simulink model "SF020_SysFaultMngt"  (R2022b)
settings: configuration reference "ASW_Configuration_Set_5ms" (kept outside this file)
settings Model: DataDictionary=SF020_SysFaultMngt.sldd  Creator=donglx1  LastModifiedBy=donglx1
settings ConfigSetRef: SourceName=ASW_Configuration_Set_5ms

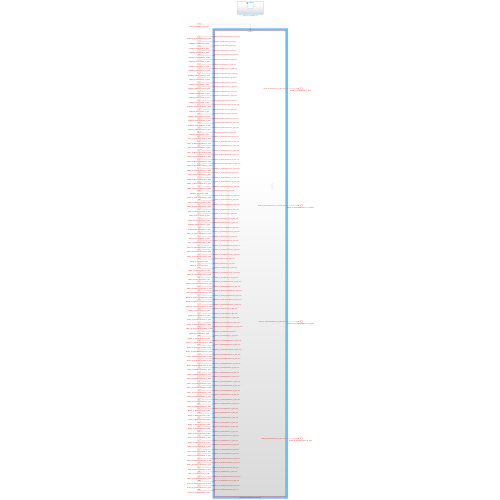
[thumbnail: Simulink's stored preview of the top-level diagram]
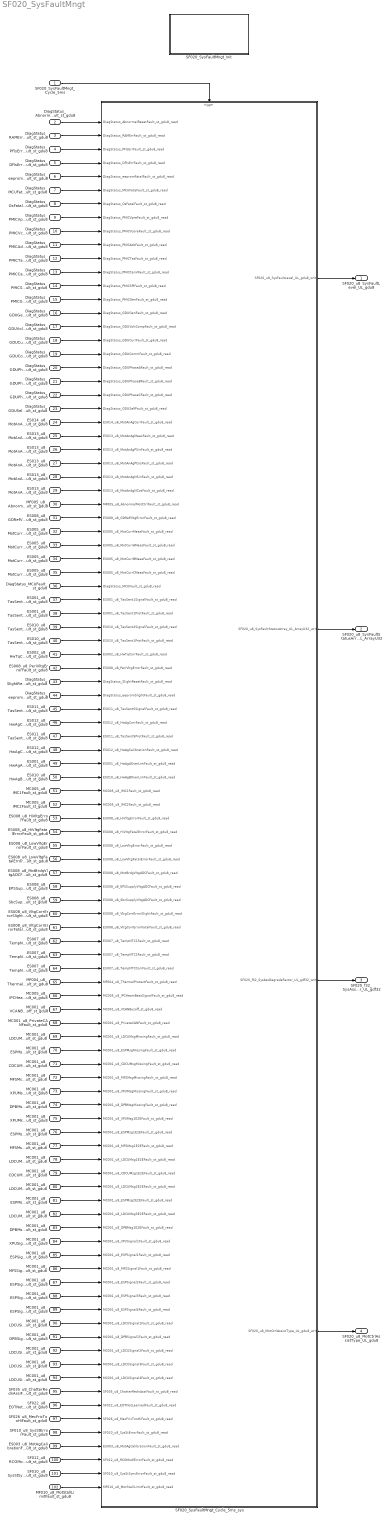
== system SF020_SysFaultMngt ==
  SF020_SysFaultMngt_Cycle_5ms : Inport  SampleTime=0.005  OutputFunctionCall=on
  DiagStatus_AbnormalResetFault_st_gdu8 : Inport  Port=2  OutDataTypeStr=UINT8  PortDimensions=1
  DiagStatus_RAMErrFault_st_gdu8 : Inport  Port=3  OutDataTypeStr=UINT8  PortDimensions=1
  DiagStatus_PFlsErrFault_st_gdu8 : Inport  Port=4  OutDataTypeStr=UINT8  PortDimensions=1
  DiagStatus_DFlsErrFault_st_gdu8 : Inport  Port=5  OutDataTypeStr=UINT8  PortDimensions=1
  DiagStatus_eepromFatalFault_st_gdu8 : Inport  Port=6  OutDataTypeStr=UINT8  PortDimensions=1
  DiagStatus_MCUFataFault_st_gdu8 : Inport  Port=7  OutDataTypeStr=UINT8  PortDimensions=1
  DiagStatus_OsFatalFault_st_gdu8 : Inport  Port=8  OutDataTypeStr=UINT8  PortDimensions=1
  DiagStatus_PMICVpreFault_st_gdu8 : Inport  Port=9  OutDataTypeStr=UINT8  PortDimensions=1
  DiagStatus_PMICVcoreFault_st_gdu8 : Inport  Port=10  OutDataTypeStr=UINT8  PortDimensions=1
  DiagStatus_PMICAdcFault_st_gdu8 : Inport  Port=11  OutDataTypeStr=UINT8  PortDimensions=1
  DiagStatus_PMICTasFault_st_gdu8 : Inport  Port=12  OutDataTypeStr=UINT8  PortDimensions=1
  DiagStatus_PMICCanVFault_st_gdu8 : Inport  Port=13  OutDataTypeStr=UINT8  PortDimensions=1
  DiagStatus_PMICSPIFault_st_gdu8 : Inport  Port=14  OutDataTypeStr=UINT8  PortDimensions=1
  DiagStatus_PMICGenFault_st_gdu8 : Inport  Port=15  OutDataTypeStr=UINT8  PortDimensions=1
  DiagStatus_GDUGenFault_st_gdu8 : Inport  Port=16  OutDataTypeStr=UINT8  PortDimensions=1
  DiagStatus_GDUVoltCompFault_st_gdu8 : Inport  Port=17  OutDataTypeStr=UINT8  PortDimensions=1
  DiagStatus_GDUCurrFault_st_gdu8 : Inport  Port=18  OutDataTypeStr=UINT8  PortDimensions=1
  DiagStatus_GDUCommFault_st_gdu8 : Inport  Port=19  OutDataTypeStr=UINT8  PortDimensions=1
  DiagStatus_GDUPhaseAFault_st_gdu8 : Inport  Port=20  OutDataTypeStr=UINT8  PortDimensions=1
  DiagStatus_GDUPhaseBFault_st_gdu8 : Inport  Port=21  OutDataTypeStr=UINT8  PortDimensions=1
  DiagStatus_GDUPhaseCFault_st_gdu8 : Inport  Port=22  OutDataTypeStr=UINT8  PortDimensions=1
  DiagStatus_GDUSelfFault_st_gdu8 : Inport  Port=23  OutDataTypeStr=UINT8  PortDimensions=1
  ES014_u8_MotAnAgCorrFault_st_gdu8 : Inport  Port=24  OutDataTypeStr=UINT8  PortDimensions=1
  ES013_u8_MotAnAgMeasFault_st_gdu8 : Inport  Port=25  OutDataTypeStr=UINT8  PortDimensions=1
  ES013_u8_MotAnAgPSinFault_st_gdu8 : Inport  Port=26  OutDataTypeStr=UINT8  PortDimensions=1
  ES013_u8_MotAnAgPCosFault_st_gdu8 : Inport  Port=27  OutDataTypeStr=UINT8  PortDimensions=1
  ES013_u8_MotAnAgNSinFault_st_gdu8 : Inport  Port=28  OutDataTypeStr=UINT8  PortDimensions=1
  ES013_u8_MotAnAgNCosFault_st_gdu8 : Inport  Port=29  OutDataTypeStr=UINT8  PortDimensions=1
  MF005_u8_AbnormalMotCtrlFault_st_gdu8 : Inport  Port=30  OutDataTypeStr=UINT8  PortDimensions=1
  ES008_u8_GDRefVltgErrorFault_st_gdu8 : Inport  Port=31  OutDataTypeStr=UINT8  PortDimensions=1
  ES005_u8_MotCurrMeasFault_st_gdu8 : Inport  Port=32  OutDataTypeStr=UINT8  PortDimensions=1
  ES005_u8_MotCurrAMeasFault_st_gdu8 : Inport  Port=33  OutDataTypeStr=UINT8  PortDimensions=1
  ES005_u8_MotCurrBMeasFault_st_gdu8 : Inport  Port=34  OutDataTypeStr=UINT8  PortDimensions=1
  ES005_u8_MotCurrCMeasFault_st_gdu8 : Inport  Port=35  OutDataTypeStr=UINT8  PortDimensions=1
  DiagStatus_MCUFault_st_gdu8 : Inport  Port=36  OutDataTypeStr=UINT8  PortDimensions=1
  ES001_u8_TasSent1SignalFault_st_gdu8 : Inport  Port=37  OutDataTypeStr=UINT8  PortDimensions=1
  ES001_u8_TasSent1ProtFault_st_gdu8 : Inport  Port=38  OutDataTypeStr=UINT8  PortDimensions=1
  ES010_u8_TasSent2SignalFault_st_gdu8 : Inport  Port=39  OutDataTypeStr=UINT8  PortDimensions=1
  ES010_u8_TasSent1ProtFault_st_gdu8 : Inport  Port=40  OutDataTypeStr=UINT8  PortDimensions=1
  ES002_u8_HwTqCorrFault_st_gdu8 : Inport  Port=41  OutDataTypeStr=UINT8  PortDimensions=1
  ES008_u8_PeriVltgErrorFault_st_gdu8 : Inport  Port=42  OutDataTypeStr=UINT8  PortDimensions=1
  DiagStatus_SlightResetFault_st_gdu8 : Inport  Port=43  OutDataTypeStr=UINT8  PortDimensions=1
  DiagStatus_eepromSlightFault_st_gdu8 : Inport  Port=44  OutDataTypeStr=UINT8  PortDimensions=1
  ES011_u8_TasSent5SignalFault_st_gdu8 : Inport  Port=45  OutDataTypeStr=UINT8  PortDimensions=1
  ES012_u8_HwAgCorrFault_st_gdu8 : Inport  Port=46  OutDataTypeStr=UINT8  PortDimensions=1
  ES011_u8_TasSent5ProtFault_st_gdu8 : Inport  Port=47  OutDataTypeStr=UINT8  PortDimensions=1
  ES012_u8_HwAgCalibrationFault_st_gdu8 : Inport  Port=48  OutDataTypeStr=UINT8  PortDimensions=1
  ES001_u8_HwAgAOverLimFault_st_gdu8 : Inport  Port=49  OutDataTypeStr=UINT8  PortDimensions=1
  ES010_u8_HwAgBOverLimFault_st_gdu8 : Inport  Port=50  OutDataTypeStr=UINT8  PortDimensions=1
  MC005_u8_IMC1Fault_st_gdu8 : Inport  Port=51  OutDataTypeStr=UINT8  PortDimensions=1
  MC005_u8_IMC2Fault_st_gdu8 : Inport  Port=52  OutDataTypeStr=UINT8  PortDimensions=1
  ES008_u8_HiVltgErrorFault_st_gdu8 : Inport  Port=53  OutDataTypeStr=UINT8  PortDimensions=1
  ES008_u8_HiVltgFatalErrorFault_st_gdu8 : Inport  Port=54  OutDataTypeStr=UINT8  PortDimensions=1
  ES008_u8_LowVltgErrorFault_st_gdu8 : Inport  Port=55  OutDataTypeStr=UINT8  PortDimensions=1
  ES008_u8_LowVltgFatalErrorFault_st_gdu8 : Inport  Port=56  OutDataTypeStr=UINT8  PortDimensions=1
  ES008_u8_MotBrdgVltgADCFault_st_gdu8 : Inport  Port=57  OutDataTypeStr=UINT8  PortDimensions=1
  ES008_u8_EPSSupplyVltgADCFault_st_gdu8 : Inport  Port=58  OutDataTypeStr=UINT8  PortDimensions=1
  ES008_u8_SbcSupplyVltgADCFault_st_gdu8 : Inport  Port=59  OutDataTypeStr=UINT8  PortDimensions=1
  ES008_u8_VltgCorrErrorSlightFault_st_gdu8 : Inport  Port=60  OutDataTypeStr=UINT8  PortDimensions=1
  ES008_u8_VltgCorrErrorFatalFault_st_gdu8 : Inport  Port=61  OutDataTypeStr=UINT8  PortDimensions=1
  ES007_u8_TempNTC1Fault_st_gdu8 : Inport  Port=62  OutDataTypeStr=UINT8  PortDimensions=1
  ES007_u8_TempNTC2Fault_st_gdu8 : Inport  Port=63  OutDataTypeStr=UINT8  PortDimensions=1
  ES007_u8_TempNTCCorrFault_st_gdu8 : Inport  Port=64  OutDataTypeStr=UINT8  PortDimensions=1
  MF004_u8_ThermalProtectFault_st_gdu8 : Inport  Port=65  OutDataTypeStr=UINT8  PortDimensions=1
  MC005_u8_IPCHeartBeatSignalFault_st_gdu8 : Inport  Port=66  OutDataTypeStr=UINT8  PortDimensions=1
  MC001_u8_VCANBusoff_st_gdu8 : Inport  Port=67  OutDataTypeStr=UINT8  PortDimensions=1
  MC001_u8_PrivateCANFault_st_gdu8 : Inport  Port=68  OutDataTypeStr=UINT8  PortDimensions=1
  MC001_u8_LDCUMsgMissingFault_st_gdu8 : Inport  Port=69  OutDataTypeStr=UINT8  PortDimensions=1
  MC001_u8_ESPMsgMissingFault_st_gdu8 : Inport  Port=70  OutDataTypeStr=UINT8  PortDimensions=1
  MC001_u8_CDCUMsgMissingFault_st_gdu8 : Inport  Port=71  OutDataTypeStr=UINT8  PortDimensions=1
  MC001_u8_MFSMsgMissingFault_st_gdu8 : Inport  Port=72  OutDataTypeStr=UINT8  PortDimensions=1
  MC001_u8_XPUMsgMissingFault_st_gdu8 : Inport  Port=73  OutDataTypeStr=UINT8  PortDimensions=1
  MC001_u8_DPBMsgMissingFault_st_gdu8 : Inport  Port=74  OutDataTypeStr=UINT8  PortDimensions=1
  MC001_u8_XPUMsg1E2EFault_st_gdu8 : Inport  Port=75  OutDataTypeStr=UINT8  PortDimensions=1
  MC001_u8_ESPMsg1E2EFault_st_gdu8 : Inport  Port=76  OutDataTypeStr=UINT8  PortDimensions=1
  MC001_u8_MFSMsg1E2EFault_st_gdu8 : Inport  Port=77  OutDataTypeStr=UINT8  PortDimensions=1
  MC001_u8_LDCUMsg1E2EFault_st_gdu8 : Inport  Port=78  OutDataTypeStr=UINT8  PortDimensions=1
  MC001_u8_CDCUMsg1E2EFault_st_gdu8 : Inport  Port=79  OutDataTypeStr=UINT8  PortDimensions=1
  MC001_u8_LDCUMsg2E2EFault_st_gdu8 : Inport  Port=80  OutDataTypeStr=UINT8  PortDimensions=1
  MC001_u8_ESPMsg2E2EFault_st_gdu8 : Inport  Port=81  OutDataTypeStr=UINT8  PortDimensions=1
  MC001_u8_LDCUMsg3E2EFault_st_gdu8 : Inport  Port=82  OutDataTypeStr=UINT8  PortDimensions=1
  MC001_u8_DPBMsg1E2EFault_st_gdu8 : Inport  Port=83  OutDataTypeStr=UINT8  PortDimensions=1
  MC001_u8_XPUSignal1Fault_st_gdu8 : Inport  Port=84  OutDataTypeStr=UINT8  PortDimensions=1
  MC001_u8_ESPSignal1Fault_st_gdu8 : Inport  Port=85  OutDataTypeStr=UINT8  PortDimensions=1
  MC001_u8_MFSSignal1Fault_st_gdu8 : Inport  Port=86  OutDataTypeStr=UINT8  PortDimensions=1
  MC001_u8_ESPSignal2Fault_st_gdu8 : Inport  Port=87  OutDataTypeStr=UINT8  PortDimensions=1
  MC001_u8_ESPSignal3Fault_st_gdu8 : Inport  Port=88  OutDataTypeStr=UINT8  PortDimensions=1
  MC001_u8_ESPSignal4Fault_st_gdu8 : Inport  Port=89  OutDataTypeStr=UINT8  PortDimensions=1
  MC001_u8_LDCUSignal1Fault_st_gdu8 : Inport  Port=90  OutDataTypeStr=UINT8  PortDimensions=1
  MC001_u8_DPBSignal1Fault_st_gdu8 : Inport  Port=91  OutDataTypeStr=UINT8  PortDimensions=1
  MC001_u8_LDCUSignal2Fault_st_gdu8 : Inport  Port=92  OutDataTypeStr=UINT8  PortDimensions=1
  MC001_u8_LDCUSignal3Fault_st_gdu8 : Inport  Port=93  OutDataTypeStr=UINT8  PortDimensions=1
  MC001_u8_LDCUSignal4Fault_st_gdu8 : Inport  Port=94  OutDataTypeStr=UINT8  PortDimensions=1
  SF035_u8_ChatterRednAssiFault_st_gdu8 : Inport  Port=95  OutDataTypeStr=UINT8  PortDimensions=1
  SF022_u8_EOTNotLearnedFault_st_gdu8 : Inport  Port=96  OutDataTypeStr=UINT8  PortDimensions=1
  SF026_u8_MecFricTooHiFault_st_gdu8 : Inport  Port=97  OutDataTypeStr=UINT8  PortDimensions=1
  SF010_u8_SysStErrorFault_st_gdu8 : Inport  Port=98  OutDataTypeStr=UINT8  PortDimensions=1
  ES003_u8_MotAgCalibrationFault_st_gdu8 : Inport  Port=99  OutDataTypeStr=UINT8  PortDimensions=1
  SF012_u8_RCOModlErrorFault_st_gdu8 : Inport  Port=100  OutDataTypeStr=UINT8  PortDimensions=1
  SF010_u8_SysStSyncErrorFault_st_gdu8 : Inport  Port=101  OutDataTypeStr=UINT8  PortDimensions=1
  MF010_u8_MotStallLimitFault_st_gdu8 : Inport  Port=102  OutDataTypeStr=UINT8  PortDimensions=1
  SF020_SysFaultMngt_Cycle_5ms_sys : Subsystem
  SF020_SysFaultMngt_Init : Subsystem
  SF020_u8_SysFaultLevel_UL_gdu8 : Outport  OutDataTypeStr=UINT8  PortDimensions=1
  SF020_u8_SysFaultStatusArray_UL_ArrayU32 : Outport  Port=2  OutDataTypeStr=UINT8  PortDimensions=32
  SF020_f32_SysAssDegradeFactor_UL_gdf32 : Outport  Port=3  OutDataTypeStr=FLOAT32  PortDimensions=1
  SF020_u8_MotCtrlAssistType_UL_gdu8 : Outport  Port=4  OutDataTypeStr=UINT8  PortDimensions=1
  wires:
  DiagStatus_AbnormalResetFault_st_gdu8/1 -> SF020_SysFaultMngt_Cycle_5ms_sys/1(DiagStatus_AbnormalResetFault_st_gdu8_read)
  DiagStatus_RAMErrFault_st_gdu8/1 -> SF020_SysFaultMngt_Cycle_5ms_sys/2(DiagStatus_RAMErrFault_st_gdu8_read)
  DiagStatus_PFlsErrFault_st_gdu8/1 -> SF020_SysFaultMngt_Cycle_5ms_sys/3(DiagStatus_PFlsErrFault_st_gdu8_read)
  DiagStatus_DFlsErrFault_st_gdu8/1 -> SF020_SysFaultMngt_Cycle_5ms_sys/4(DiagStatus_DFlsErrFault_st_gdu8_read)
  DiagStatus_eepromFatalFault_st_gdu8/1 -> SF020_SysFaultMngt_Cycle_5ms_sys/5(DiagStatus_eepromFatalFault_st_gdu8_read)
  DiagStatus_MCUFataFault_st_gdu8/1 -> SF020_SysFaultMngt_Cycle_5ms_sys/6(DiagStatus_MCUFataFault_st_gdu8_read)
  DiagStatus_OsFatalFault_st_gdu8/1 -> SF020_SysFaultMngt_Cycle_5ms_sys/7(DiagStatus_OsFatalFault_st_gdu8_read)
  DiagStatus_PMICVpreFault_st_gdu8/1 -> SF020_SysFaultMngt_Cycle_5ms_sys/8(DiagStatus_PMICVpreFault_st_gdu8_read)
  DiagStatus_PMICVcoreFault_st_gdu8/1 -> SF020_SysFaultMngt_Cycle_5ms_sys/9(DiagStatus_PMICVcoreFault_st_gdu8_read)
  DiagStatus_PMICAdcFault_st_gdu8/1 -> SF020_SysFaultMngt_Cycle_5ms_sys/10(DiagStatus_PMICAdcFault_st_gdu8_read)
  DiagStatus_PMICTasFault_st_gdu8/1 -> SF020_SysFaultMngt_Cycle_5ms_sys/11(DiagStatus_PMICTasFault_st_gdu8_read)
  DiagStatus_PMICCanVFault_st_gdu8/1 -> SF020_SysFaultMngt_Cycle_5ms_sys/12(DiagStatus_PMICCanVFault_st_gdu8_read)
  DiagStatus_PMICSPIFault_st_gdu8/1 -> SF020_SysFaultMngt_Cycle_5ms_sys/13(DiagStatus_PMICSPIFault_st_gdu8_read)
  DiagStatus_PMICGenFault_st_gdu8/1 -> SF020_SysFaultMngt_Cycle_5ms_sys/14(DiagStatus_PMICGenFault_st_gdu8_read)
  DiagStatus_GDUGenFault_st_gdu8/1 -> SF020_SysFaultMngt_Cycle_5ms_sys/15(DiagStatus_GDUGenFault_st_gdu8_read)
  DiagStatus_GDUVoltCompFault_st_gdu8/1 -> SF020_SysFaultMngt_Cycle_5ms_sys/16(DiagStatus_GDUVoltCompFault_st_gdu8_read)
  DiagStatus_GDUCurrFault_st_gdu8/1 -> SF020_SysFaultMngt_Cycle_5ms_sys/17(DiagStatus_GDUCurrFault_st_gdu8_read)
  DiagStatus_GDUCommFault_st_gdu8/1 -> SF020_SysFaultMngt_Cycle_5ms_sys/18(DiagStatus_GDUCommFault_st_gdu8_read)
  DiagStatus_GDUPhaseAFault_st_gdu8/1 -> SF020_SysFaultMngt_Cycle_5ms_sys/19(DiagStatus_GDUPhaseAFault_st_gdu8_read)
  DiagStatus_GDUPhaseBFault_st_gdu8/1 -> SF020_SysFaultMngt_Cycle_5ms_sys/20(DiagStatus_GDUPhaseBFault_st_gdu8_read)
  DiagStatus_GDUPhaseCFault_st_gdu8/1 -> SF020_SysFaultMngt_Cycle_5ms_sys/21(DiagStatus_GDUPhaseCFault_st_gdu8_read)
  DiagStatus_GDUSelfFault_st_gdu8/1 -> SF020_SysFaultMngt_Cycle_5ms_sys/22(DiagStatus_GDUSelfFault_st_gdu8_read)
  ES014_u8_MotAnAgCorrFault_st_gdu8/1 -> SF020_SysFaultMngt_Cycle_5ms_sys/23(ES014_u8_MotAnAgCorrFault_st_gdu8_read)
  ES013_u8_MotAnAgMeasFault_st_gdu8/1 -> SF020_SysFaultMngt_Cycle_5ms_sys/24(ES013_u8_MotAnAgMeasFault_st_gdu8_read)
  ES013_u8_MotAnAgPSinFault_st_gdu8/1 -> SF020_SysFaultMngt_Cycle_5ms_sys/25(ES013_u8_MotAnAgPSinFault_st_gdu8_read)
  ES013_u8_MotAnAgPCosFault_st_gdu8/1 -> SF020_SysFaultMngt_Cycle_5ms_sys/26(ES013_u8_MotAnAgPCosFault_st_gdu8_read)
  ES013_u8_MotAnAgNSinFault_st_gdu8/1 -> SF020_SysFaultMngt_Cycle_5ms_sys/27(ES013_u8_MotAnAgNSinFault_st_gdu8_read)
  ES013_u8_MotAnAgNCosFault_st_gdu8/1 -> SF020_SysFaultMngt_Cycle_5ms_sys/28(ES013_u8_MotAnAgNCosFault_st_gdu8_read)
  MF005_u8_AbnormalMotCtrlFault_st_gdu8/1 -> SF020_SysFaultMngt_Cycle_5ms_sys/29(MF005_u8_AbnormalMotCtrlFault_st_gdu8_read)
  ES008_u8_GDRefVltgErrorFault_st_gdu8/1 -> SF020_SysFaultMngt_Cycle_5ms_sys/30(ES008_u8_GDRefVltgErrorFault_st_gdu8_read)
  ES005_u8_MotCurrMeasFault_st_gdu8/1 -> SF020_SysFaultMngt_Cycle_5ms_sys/31(ES005_u8_MotCurrMeasFault_st_gdu8_read)
  ES005_u8_MotCurrAMeasFault_st_gdu8/1 -> SF020_SysFaultMngt_Cycle_5ms_sys/32(ES005_u8_MotCurrAMeasFault_st_gdu8_read)
  ES005_u8_MotCurrBMeasFault_st_gdu8/1 -> SF020_SysFaultMngt_Cycle_5ms_sys/33(ES005_u8_MotCurrBMeasFault_st_gdu8_read)
  ES005_u8_MotCurrCMeasFault_st_gdu8/1 -> SF020_SysFaultMngt_Cycle_5ms_sys/34(ES005_u8_MotCurrCMeasFault_st_gdu8_read)
  DiagStatus_MCUFault_st_gdu8/1 -> SF020_SysFaultMngt_Cycle_5ms_sys/35(DiagStatus_MCUFault_st_gdu8_read)
  ES001_u8_TasSent1SignalFault_st_gdu8/1 -> SF020_SysFaultMngt_Cycle_5ms_sys/36(ES001_u8_TasSent1SignalFault_st_gdu8_read)
  ES001_u8_TasSent1ProtFault_st_gdu8/1 -> SF020_SysFaultMngt_Cycle_5ms_sys/37(ES001_u8_TasSent1ProtFault_st_gdu8_read)
  ES010_u8_TasSent2SignalFault_st_gdu8/1 -> SF020_SysFaultMngt_Cycle_5ms_sys/38(ES010_u8_TasSent2SignalFault_st_gdu8_read)
  ES010_u8_TasSent1ProtFault_st_gdu8/1 -> SF020_SysFaultMngt_Cycle_5ms_sys/39(ES010_u8_TasSent1ProtFault_st_gdu8_read)
  ES002_u8_HwTqCorrFault_st_gdu8/1 -> SF020_SysFaultMngt_Cycle_5ms_sys/40(ES002_u8_HwTqCorrFault_st_gdu8_read)
  ES008_u8_PeriVltgErrorFault_st_gdu8/1 -> SF020_SysFaultMngt_Cycle_5ms_sys/41(ES008_u8_PeriVltgErrorFault_st_gdu8_read)
  DiagStatus_SlightResetFault_st_gdu8/1 -> SF020_SysFaultMngt_Cycle_5ms_sys/42(DiagStatus_SlightResetFault_st_gdu8_read)
  DiagStatus_eepromSlightFault_st_gdu8/1 -> SF020_SysFaultMngt_Cycle_5ms_sys/43(DiagStatus_eepromSlightFault_st_gdu8_read)
  ES011_u8_TasSent5SignalFault_st_gdu8/1 -> SF020_SysFaultMngt_Cycle_5ms_sys/44(ES011_u8_TasSent5SignalFault_st_gdu8_read)
  ES012_u8_HwAgCorrFault_st_gdu8/1 -> SF020_SysFaultMngt_Cycle_5ms_sys/45(ES012_u8_HwAgCorrFault_st_gdu8_read)
  ES011_u8_TasSent5ProtFault_st_gdu8/1 -> SF020_SysFaultMngt_Cycle_5ms_sys/46(ES011_u8_TasSent5ProtFault_st_gdu8_read)
  ES012_u8_HwAgCalibrationFault_st_gdu8/1 -> SF020_SysFaultMngt_Cycle_5ms_sys/47(ES012_u8_HwAgCalibrationFault_st_gdu8_read)
  ES001_u8_HwAgAOverLimFault_st_gdu8/1 -> SF020_SysFaultMngt_Cycle_5ms_sys/48(ES001_u8_HwAgAOverLimFault_st_gdu8_read)
  ES010_u8_HwAgBOverLimFault_st_gdu8/1 -> SF020_SysFaultMngt_Cycle_5ms_sys/49(ES010_u8_HwAgBOverLimFault_st_gdu8_read)
  MC005_u8_IMC1Fault_st_gdu8/1 -> SF020_SysFaultMngt_Cycle_5ms_sys/50(MC005_u8_IMC1Fault_st_gdu8_read)
  MC005_u8_IMC2Fault_st_gdu8/1 -> SF020_SysFaultMngt_Cycle_5ms_sys/51(MC005_u8_IMC2Fault_st_gdu8_read)
  ES008_u8_HiVltgErrorFault_st_gdu8/1 -> SF020_SysFaultMngt_Cycle_5ms_sys/52(ES008_u8_HiVltgErrorFault_st_gdu8_read)
  ES008_u8_HiVltgFatalErrorFault_st_gdu8/1 -> SF020_SysFaultMngt_Cycle_5ms_sys/53(ES008_u8_HiVltgFatalErrorFault_st_gdu8_read)
  ES008_u8_LowVltgErrorFault_st_gdu8/1 -> SF020_SysFaultMngt_Cycle_5ms_sys/54(ES008_u8_LowVltgErrorFault_st_gdu8_read)
  ES008_u8_LowVltgFatalErrorFault_st_gdu8/1 -> SF020_SysFaultMngt_Cycle_5ms_sys/55(ES008_u8_LowVltgFatalErrorFault_st_gdu8_read)
  ES008_u8_MotBrdgVltgADCFault_st_gdu8/1 -> SF020_SysFaultMngt_Cycle_5ms_sys/56(ES008_u8_MotBrdgVltgADCFault_st_gdu8_read)
  ES008_u8_EPSSupplyVltgADCFault_st_gdu8/1 -> SF020_SysFaultMngt_Cycle_5ms_sys/57(ES008_u8_EPSSupplyVltgADCFault_st_gdu8_read)
  ES008_u8_SbcSupplyVltgADCFault_st_gdu8/1 -> SF020_SysFaultMngt_Cycle_5ms_sys/58(ES008_u8_SbcSupplyVltgADCFault_st_gdu8_read)
  ES008_u8_VltgCorrErrorSlightFault_st_gdu8/1 -> SF020_SysFaultMngt_Cycle_5ms_sys/59(ES008_u8_VltgCorrErrorSlightFault_st_gdu8_read)
  ES008_u8_VltgCorrErrorFatalFault_st_gdu8/1 -> SF020_SysFaultMngt_Cycle_5ms_sys/60(ES008_u8_VltgCorrErrorFatalFault_st_gdu8_read)
  ES007_u8_TempNTC1Fault_st_gdu8/1 -> SF020_SysFaultMngt_Cycle_5ms_sys/61(ES007_u8_TempNTC1Fault_st_gdu8_read)
  ES007_u8_TempNTC2Fault_st_gdu8/1 -> SF020_SysFaultMngt_Cycle_5ms_sys/62(ES007_u8_TempNTC2Fault_st_gdu8_read)
  ES007_u8_TempNTCCorrFault_st_gdu8/1 -> SF020_SysFaultMngt_Cycle_5ms_sys/63(ES007_u8_TempNTCCorrFault_st_gdu8_read)
  MF004_u8_ThermalProtectFault_st_gdu8/1 -> SF020_SysFaultMngt_Cycle_5ms_sys/64(MF004_u8_ThermalProtectFault_st_gdu8_read)
  MC005_u8_IPCHeartBeatSignalFault_st_gdu8/1 -> SF020_SysFaultMngt_Cycle_5ms_sys/65(MC005_u8_IPCHeartBeatSignalFault_st_gdu8_read)
  MC001_u8_VCANBusoff_st_gdu8/1 -> SF020_SysFaultMngt_Cycle_5ms_sys/66(MC001_u8_VCANBusoff_st_gdu8_read)
  MC001_u8_PrivateCANFault_st_gdu8/1 -> SF020_SysFaultMngt_Cycle_5ms_sys/67(MC001_u8_PrivateCANFault_st_gdu8_read)
  MC001_u8_LDCUMsgMissingFault_st_gdu8/1 -> SF020_SysFaultMngt_Cycle_5ms_sys/68(MC001_u8_LDCUMsgMissingFault_st_gdu8_read)
  MC001_u8_ESPMsgMissingFault_st_gdu8/1 -> SF020_SysFaultMngt_Cycle_5ms_sys/69(MC001_u8_ESPMsgMissingFault_st_gdu8_read)
  MC001_u8_CDCUMsgMissingFault_st_gdu8/1 -> SF020_SysFaultMngt_Cycle_5ms_sys/70(MC001_u8_CDCUMsgMissingFault_st_gdu8_read)
  MC001_u8_MFSMsgMissingFault_st_gdu8/1 -> SF020_SysFaultMngt_Cycle_5ms_sys/71(MC001_u8_MFSMsgMissingFault_st_gdu8_read)
  MC001_u8_XPUMsgMissingFault_st_gdu8/1 -> SF020_SysFaultMngt_Cycle_5ms_sys/72(MC001_u8_XPUMsgMissingFault_st_gdu8_read)
  MC001_u8_DPBMsgMissingFault_st_gdu8/1 -> SF020_SysFaultMngt_Cycle_5ms_sys/73(MC001_u8_DPBMsgMissingFault_st_gdu8_read)
  MC001_u8_XPUMsg1E2EFault_st_gdu8/1 -> SF020_SysFaultMngt_Cycle_5ms_sys/74(MC001_u8_XPUMsg1E2EFault_st_gdu8_read)
  MC001_u8_ESPMsg1E2EFault_st_gdu8/1 -> SF020_SysFaultMngt_Cycle_5ms_sys/75(MC001_u8_ESPMsg1E2EFault_st_gdu8_read)
  MC001_u8_MFSMsg1E2EFault_st_gdu8/1 -> SF020_SysFaultMngt_Cycle_5ms_sys/76(MC001_u8_MFSMsg1E2EFault_st_gdu8_read)
  MC001_u8_LDCUMsg1E2EFault_st_gdu8/1 -> SF020_SysFaultMngt_Cycle_5ms_sys/77(MC001_u8_LDCUMsg1E2EFault_st_gdu8_read)
  MC001_u8_CDCUMsg1E2EFault_st_gdu8/1 -> SF020_SysFaultMngt_Cycle_5ms_sys/78(MC001_u8_CDCUMsg1E2EFault_st_gdu8_read)
  MC001_u8_LDCUMsg2E2EFault_st_gdu8/1 -> SF020_SysFaultMngt_Cycle_5ms_sys/79(MC001_u8_LDCUMsg2E2EFault_st_gdu8_read)
  MC001_u8_ESPMsg2E2EFault_st_gdu8/1 -> SF020_SysFaultMngt_Cycle_5ms_sys/80(MC001_u8_ESPMsg2E2EFault_st_gdu8_read)
  MC001_u8_LDCUMsg3E2EFault_st_gdu8/1 -> SF020_SysFaultMngt_Cycle_5ms_sys/81(MC001_u8_LDCUMsg3E2EFault_st_gdu8_read)
  MC001_u8_DPBMsg1E2EFault_st_gdu8/1 -> SF020_SysFaultMngt_Cycle_5ms_sys/82(MC001_u8_DPBMsg1E2EFault_st_gdu8_read)
  MC001_u8_XPUSignal1Fault_st_gdu8/1 -> SF020_SysFaultMngt_Cycle_5ms_sys/83(MC001_u8_XPUSignal1Fault_st_gdu8_read)
  MC001_u8_ESPSignal1Fault_st_gdu8/1 -> SF020_SysFaultMngt_Cycle_5ms_sys/84(MC001_u8_ESPSignal1Fault_st_gdu8_read)
  MC001_u8_MFSSignal1Fault_st_gdu8/1 -> SF020_SysFaultMngt_Cycle_5ms_sys/85(MC001_u8_MFSSignal1Fault_st_gdu8_read)
  MC001_u8_ESPSignal2Fault_st_gdu8/1 -> SF020_SysFaultMngt_Cycle_5ms_sys/86(MC001_u8_ESPSignal2Fault_st_gdu8_read)
  MC001_u8_ESPSignal3Fault_st_gdu8/1 -> SF020_SysFaultMngt_Cycle_5ms_sys/87(MC001_u8_ESPSignal3Fault_st_gdu8_read)
  MC001_u8_ESPSignal4Fault_st_gdu8/1 -> SF020_SysFaultMngt_Cycle_5ms_sys/88(MC001_u8_ESPSignal4Fault_st_gdu8_read)
  MC001_u8_LDCUSignal1Fault_st_gdu8/1 -> SF020_SysFaultMngt_Cycle_5ms_sys/89(MC001_u8_LDCUSignal1Fault_st_gdu8_read)
  MC001_u8_DPBSignal1Fault_st_gdu8/1 -> SF020_SysFaultMngt_Cycle_5ms_sys/90(MC001_u8_DPBSignal1Fault_st_gdu8_read)
  MC001_u8_LDCUSignal2Fault_st_gdu8/1 -> SF020_SysFaultMngt_Cycle_5ms_sys/91(MC001_u8_LDCUSignal2Fault_st_gdu8_read)
  MC001_u8_LDCUSignal3Fault_st_gdu8/1 -> SF020_SysFaultMngt_Cycle_5ms_sys/92(MC001_u8_LDCUSignal3Fault_st_gdu8_read)
  MC001_u8_LDCUSignal4Fault_st_gdu8/1 -> SF020_SysFaultMngt_Cycle_5ms_sys/93(MC001_u8_LDCUSignal4Fault_st_gdu8_read)
  SF035_u8_ChatterRednAssiFault_st_gdu8/1 -> SF020_SysFaultMngt_Cycle_5ms_sys/94(SF035_u8_ChatterRednAssiFault_st_gdu8_read)
  SF022_u8_EOTNotLearnedFault_st_gdu8/1 -> SF020_SysFaultMngt_Cycle_5ms_sys/95(SF022_u8_EOTNotLearnedFault_st_gdu8_read)
  SF026_u8_MecFricTooHiFault_st_gdu8/1 -> SF020_SysFaultMngt_Cycle_5ms_sys/96(SF026_u8_MecFricTooHiFault_st_gdu8_read)
  SF010_u8_SysStErrorFault_st_gdu8/1 -> SF020_SysFaultMngt_Cycle_5ms_sys/97(SF010_u8_SysStErrorFault_st_gdu8_read)
  ES003_u8_MotAgCalibrationFault_st_gdu8/1 -> SF020_SysFaultMngt_Cycle_5ms_sys/98(ES003_u8_MotAgCalibrationFault_st_gdu8_read)
  SF012_u8_RCOModlErrorFault_st_gdu8/1 -> SF020_SysFaultMngt_Cycle_5ms_sys/99(SF012_u8_RCOModlErrorFault_st_gdu8_read)
  SF010_u8_SysStSyncErrorFault_st_gdu8/1 -> SF020_SysFaultMngt_Cycle_5ms_sys/100(SF010_u8_SysStSyncErrorFault_st_gdu8_read)
  MF010_u8_MotStallLimitFault_st_gdu8/1 -> SF020_SysFaultMngt_Cycle_5ms_sys/101(MF010_u8_MotStallLimitFault_st_gdu8_read)
  SF020_SysFaultMngt_Cycle_5ms_sys/1(SF020_u8_SysFaultLevel_UL_gdu8_write) -> SF020_u8_SysFaultLevel_UL_gdu8/1
  SF020_SysFaultMngt_Cycle_5ms_sys/2(SF020_u8_SysFaultStatusArray_UL_ArrayU32_write) -> SF020_u8_SysFaultStatusArray_UL_ArrayU32/1
  SF020_SysFaultMngt_Cycle_5ms_sys/3(SF020_f32_SysAssDegradeFactor_UL_gdf32_write) -> SF020_f32_SysAssDegradeFactor_UL_gdf32/1
  SF020_SysFaultMngt_Cycle_5ms_sys/4(SF020_u8_MotCtrlAssistType_UL_gdu8_write) -> SF020_u8_MotCtrlAssistType_UL_gdu8/1
  SF020_SysFaultMngt_Cycle_5ms/1 -> SF020_SysFaultMngt_Cycle_5ms_sys/Trigger

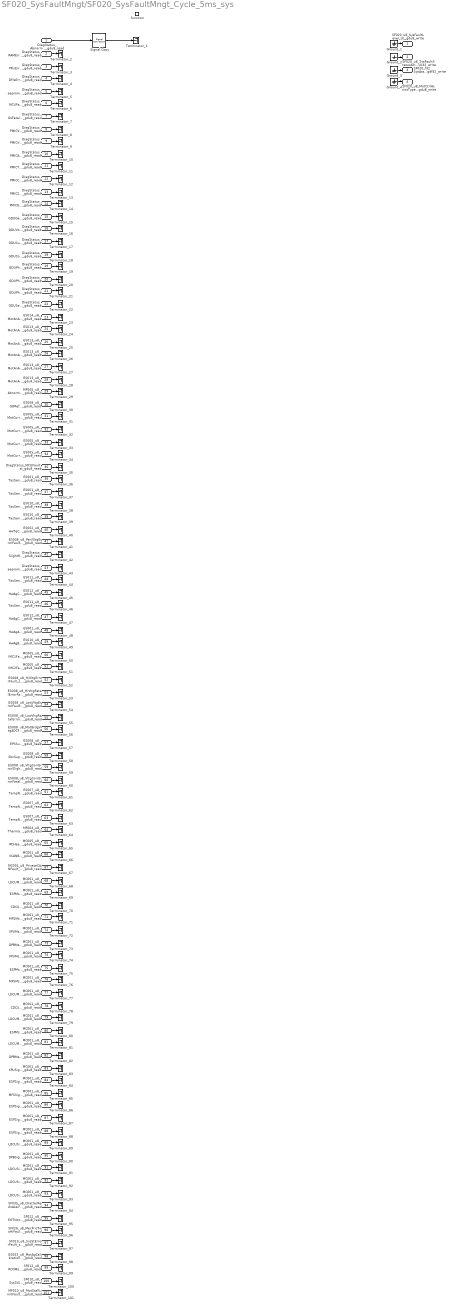
== system SF020_SysFaultMngt/SF020_SysFaultMngt_Cycle_5ms_sys ==
  DiagStatus_AbnormalResetFault_st_gdu8_read : Inport
  DiagStatus_RAMErrFault_st_gdu8_read : Inport  Port=2
  DiagStatus_PFlsErrFault_st_gdu8_read : Inport  Port=3
  DiagStatus_DFlsErrFault_st_gdu8_read : Inport  Port=4
  DiagStatus_eepromFatalFault_st_gdu8_read : Inport  Port=5
  DiagStatus_MCUFataFault_st_gdu8_read : Inport  Port=6
  DiagStatus_OsFatalFault_st_gdu8_read : Inport  Port=7
  DiagStatus_PMICVpreFault_st_gdu8_read : Inport  Port=8
  DiagStatus_PMICVcoreFault_st_gdu8_read : Inport  Port=9
  DiagStatus_PMICAdcFault_st_gdu8_read : Inport  Port=10
  DiagStatus_PMICTasFault_st_gdu8_read : Inport  Port=11
  DiagStatus_PMICCanVFault_st_gdu8_read : Inport  Port=12
  DiagStatus_PMICSPIFault_st_gdu8_read : Inport  Port=13
  DiagStatus_PMICGenFault_st_gdu8_read : Inport  Port=14
  DiagStatus_GDUGenFault_st_gdu8_read : Inport  Port=15
  DiagStatus_GDUVoltCompFault_st_gdu8_read : Inport  Port=16
  DiagStatus_GDUCurrFault_st_gdu8_read : Inport  Port=17
  DiagStatus_GDUCommFault_st_gdu8_read : Inport  Port=18
  DiagStatus_GDUPhaseAFault_st_gdu8_read : Inport  Port=19
  DiagStatus_GDUPhaseBFault_st_gdu8_read : Inport  Port=20
  DiagStatus_GDUPhaseCFault_st_gdu8_read : Inport  Port=21
  DiagStatus_GDUSelfFault_st_gdu8_read : Inport  Port=22
  ES014_u8_MotAnAgCorrFault_st_gdu8_read : Inport  Port=23
  ES013_u8_MotAnAgMeasFault_st_gdu8_read : Inport  Port=24
  ES013_u8_MotAnAgPSinFault_st_gdu8_read : Inport  Port=25
  ES013_u8_MotAnAgPCosFault_st_gdu8_read : Inport  Port=26
  ES013_u8_MotAnAgNSinFault_st_gdu8_read : Inport  Port=27
  ES013_u8_MotAnAgNCosFault_st_gdu8_read : Inport  Port=28
  MF005_u8_AbnormalMotCtrlFault_st_gdu8_read : Inport  Port=29
  ES008_u8_GDRefVltgErrorFault_st_gdu8_read : Inport  Port=30
  ES005_u8_MotCurrMeasFault_st_gdu8_read : Inport  Port=31
  ES005_u8_MotCurrAMeasFault_st_gdu8_read : Inport  Port=32
  ES005_u8_MotCurrBMeasFault_st_gdu8_read : Inport  Port=33
  ES005_u8_MotCurrCMeasFault_st_gdu8_read : Inport  Port=34
  DiagStatus_MCUFault_st_gdu8_read : Inport  Port=35
  ES001_u8_TasSent1SignalFault_st_gdu8_read : Inport  Port=36
  ES001_u8_TasSent1ProtFault_st_gdu8_read : Inport  Port=37
  ES010_u8_TasSent2SignalFault_st_gdu8_read : Inport  Port=38
  ES010_u8_TasSent1ProtFault_st_gdu8_read : Inport  Port=39
  ES002_u8_HwTqCorrFault_st_gdu8_read : Inport  Port=40
  ES008_u8_PeriVltgErrorFault_st_gdu8_read : Inport  Port=41
  DiagStatus_SlightResetFault_st_gdu8_read : Inport  Port=42
  DiagStatus_eepromSlightFault_st_gdu8_read : Inport  Port=43
  ES011_u8_TasSent5SignalFault_st_gdu8_read : Inport  Port=44
  ES012_u8_HwAgCorrFault_st_gdu8_read : Inport  Port=45
  ES011_u8_TasSent5ProtFault_st_gdu8_read : Inport  Port=46
  ES012_u8_HwAgCalibrationFault_st_gdu8_read : Inport  Port=47
  ES001_u8_HwAgAOverLimFault_st_gdu8_read : Inport  Port=48
  ES010_u8_HwAgBOverLimFault_st_gdu8_read : Inport  Port=49
  MC005_u8_IMC1Fault_st_gdu8_read : Inport  Port=50
  MC005_u8_IMC2Fault_st_gdu8_read : Inport  Port=51
  ES008_u8_HiVltgErrorFault_st_gdu8_read : Inport  Port=52
  ES008_u8_HiVltgFatalErrorFault_st_gdu8_read : Inport  Port=53
  ES008_u8_LowVltgErrorFault_st_gdu8_read : Inport  Port=54
  ES008_u8_LowVltgFatalErrorFault_st_gdu8_read : Inport  Port=55
  ES008_u8_MotBrdgVltgADCFault_st_gdu8_read : Inport  Port=56
  ES008_u8_EPSSupplyVltgADCFault_st_gdu8_read : Inport  Port=57
  ES008_u8_SbcSupplyVltgADCFault_st_gdu8_read : Inport  Port=58
  ES008_u8_VltgCorrErrorSlightFault_st_gdu8_read : Inport  Port=59
  ES008_u8_VltgCorrErrorFatalFault_st_gdu8_read : Inport  Port=60
  ES007_u8_TempNTC1Fault_st_gdu8_read : Inport  Port=61
  ES007_u8_TempNTC2Fault_st_gdu8_read : Inport  Port=62
  ES007_u8_TempNTCCorrFault_st_gdu8_read : Inport  Port=63
  MF004_u8_ThermalProtectFault_st_gdu8_read : Inport  Port=64
  MC005_u8_IPCHeartBeatSignalFault_st_gdu8_read : Inport  Port=65
  MC001_u8_VCANBusoff_st_gdu8_read : Inport  Port=66
  MC001_u8_PrivateCANFault_st_gdu8_read : Inport  Port=67
  MC001_u8_LDCUMsgMissingFault_st_gdu8_read : Inport  Port=68
  MC001_u8_ESPMsgMissingFault_st_gdu8_read : Inport  Port=69
  MC001_u8_CDCUMsgMissingFault_st_gdu8_read : Inport  Port=70
  MC001_u8_MFSMsgMissingFault_st_gdu8_read : Inport  Port=71
  MC001_u8_XPUMsgMissingFault_st_gdu8_read : Inport  Port=72
  MC001_u8_DPBMsgMissingFault_st_gdu8_read : Inport  Port=73
  MC001_u8_XPUMsg1E2EFault_st_gdu8_read : Inport  Port=74
  MC001_u8_ESPMsg1E2EFault_st_gdu8_read : Inport  Port=75
  MC001_u8_MFSMsg1E2EFault_st_gdu8_read : Inport  Port=76
  MC001_u8_LDCUMsg1E2EFault_st_gdu8_read : Inport  Port=77
  MC001_u8_CDCUMsg1E2EFault_st_gdu8_read : Inport  Port=78
  MC001_u8_LDCUMsg2E2EFault_st_gdu8_read : Inport  Port=79
  MC001_u8_ESPMsg2E2EFault_st_gdu8_read : Inport  Port=80
  MC001_u8_LDCUMsg3E2EFault_st_gdu8_read : Inport  Port=81
  MC001_u8_DPBMsg1E2EFault_st_gdu8_read : Inport  Port=82
  MC001_u8_XPUSignal1Fault_st_gdu8_read : Inport  Port=83
  MC001_u8_ESPSignal1Fault_st_gdu8_read : Inport  Port=84
  MC001_u8_MFSSignal1Fault_st_gdu8_read : Inport  Port=85
  MC001_u8_ESPSignal2Fault_st_gdu8_read : Inport  Port=86
  MC001_u8_ESPSignal3Fault_st_gdu8_read : Inport  Port=87
  MC001_u8_ESPSignal4Fault_st_gdu8_read : Inport  Port=88
  MC001_u8_LDCUSignal1Fault_st_gdu8_read : Inport  Port=89
  MC001_u8_DPBSignal1Fault_st_gdu8_read : Inport  Port=90
  MC001_u8_LDCUSignal2Fault_st_gdu8_read : Inport  Port=91
  MC001_u8_LDCUSignal3Fault_st_gdu8_read : Inport  Port=92
  MC001_u8_LDCUSignal4Fault_st_gdu8_read : Inport  Port=93
  SF035_u8_ChatterRednAssiFault_st_gdu8_read : Inport  Port=94
  SF022_u8_EOTNotLearnedFault_st_gdu8_read : Inport  Port=95
  SF026_u8_MecFricTooHiFault_st_gdu8_read : Inport  Port=96
  SF010_u8_SysStErrorFault_st_gdu8_read : Inport  Port=97
  ES003_u8_MotAgCalibrationFault_st_gdu8_read : Inport  Port=98
  SF012_u8_RCOModlErrorFault_st_gdu8_read : Inport  Port=99
  SF010_u8_SysStSyncErrorFault_st_gdu8_read : Inport  Port=100
  MF010_u8_MotStallLimitFault_st_gdu8_read : Inport  Port=101
  function : TriggerPort  TriggerType=function-call  VariantControl=(inherit)  SampleTimeType=periodic  SampleTime=-1
  Ground_{1..4} (4 alike) : Ground
  Signal Copy : SignalConversion  OverrideOpt=off
  Terminator_{1..101} (101 alike) : Terminator
  SF020_u8_SysFaultLevel_UL_gdu8_write : Outport
      settings: EnsureOutportIsVirtual=on
  SF020_u8_SysFaultStatusArray_UL_ArrayU32_write : Outport  Port=2
      settings: EnsureOutportIsVirtual=on
  SF020_f32_SysAssDegradeFactor_UL_gdf32_write : Outport  Port=3
      settings: EnsureOutportIsVirtual=on
  SF020_u8_MotCtrlAssistType_UL_gdu8_write : Outport  Port=4
      settings: EnsureOutportIsVirtual=on
  wires:
  DiagStatus_AbnormalResetFault_st_gdu8_read/1 -> Signal Copy/1
  DiagStatus_RAMErrFault_st_gdu8_read/1 -> Terminator_2/1
  DiagStatus_PFlsErrFault_st_gdu8_read/1 -> Terminator_3/1
  DiagStatus_DFlsErrFault_st_gdu8_read/1 -> Terminator_4/1
  DiagStatus_eepromFatalFault_st_gdu8_read/1 -> Terminator_5/1
  DiagStatus_MCUFataFault_st_gdu8_read/1 -> Terminator_6/1
  DiagStatus_OsFatalFault_st_gdu8_read/1 -> Terminator_7/1
  DiagStatus_PMICVpreFault_st_gdu8_read/1 -> Terminator_8/1
  DiagStatus_PMICVcoreFault_st_gdu8_read/1 -> Terminator_9/1
  DiagStatus_PMICAdcFault_st_gdu8_read/1 -> Terminator_10/1
  DiagStatus_PMICTasFault_st_gdu8_read/1 -> Terminator_11/1
  DiagStatus_PMICCanVFault_st_gdu8_read/1 -> Terminator_12/1
  DiagStatus_PMICSPIFault_st_gdu8_read/1 -> Terminator_13/1
  DiagStatus_PMICGenFault_st_gdu8_read/1 -> Terminator_14/1
  DiagStatus_GDUGenFault_st_gdu8_read/1 -> Terminator_15/1
  DiagStatus_GDUVoltCompFault_st_gdu8_read/1 -> Terminator_16/1
  DiagStatus_GDUCurrFault_st_gdu8_read/1 -> Terminator_17/1
  DiagStatus_GDUCommFault_st_gdu8_read/1 -> Terminator_18/1
  DiagStatus_GDUPhaseAFault_st_gdu8_read/1 -> Terminator_19/1
  DiagStatus_GDUPhaseBFault_st_gdu8_read/1 -> Terminator_20/1
  DiagStatus_GDUPhaseCFault_st_gdu8_read/1 -> Terminator_21/1
  DiagStatus_GDUSelfFault_st_gdu8_read/1 -> Terminator_22/1
  ES014_u8_MotAnAgCorrFault_st_gdu8_read/1 -> Terminator_23/1
  ES013_u8_MotAnAgMeasFault_st_gdu8_read/1 -> Terminator_24/1
  ES013_u8_MotAnAgPSinFault_st_gdu8_read/1 -> Terminator_25/1
  ES013_u8_MotAnAgPCosFault_st_gdu8_read/1 -> Terminator_26/1
  ES013_u8_MotAnAgNSinFault_st_gdu8_read/1 -> Terminator_27/1
  ES013_u8_MotAnAgNCosFault_st_gdu8_read/1 -> Terminator_28/1
  MF005_u8_AbnormalMotCtrlFault_st_gdu8_read/1 -> Terminator_29/1
  ES008_u8_GDRefVltgErrorFault_st_gdu8_read/1 -> Terminator_30/1
  ES005_u8_MotCurrMeasFault_st_gdu8_read/1 -> Terminator_31/1
  ES005_u8_MotCurrAMeasFault_st_gdu8_read/1 -> Terminator_32/1
  ES005_u8_MotCurrBMeasFault_st_gdu8_read/1 -> Terminator_33/1
  ES005_u8_MotCurrCMeasFault_st_gdu8_read/1 -> Terminator_34/1
  DiagStatus_MCUFault_st_gdu8_read/1 -> Terminator_35/1
  ES001_u8_TasSent1SignalFault_st_gdu8_read/1 -> Terminator_36/1
  ES001_u8_TasSent1ProtFault_st_gdu8_read/1 -> Terminator_37/1
  ES010_u8_TasSent2SignalFault_st_gdu8_read/1 -> Terminator_38/1
  ES010_u8_TasSent1ProtFault_st_gdu8_read/1 -> Terminator_39/1
  ES002_u8_HwTqCorrFault_st_gdu8_read/1 -> Terminator_40/1
  ES008_u8_PeriVltgErrorFault_st_gdu8_read/1 -> Terminator_41/1
  DiagStatus_SlightResetFault_st_gdu8_read/1 -> Terminator_42/1
  DiagStatus_eepromSlightFault_st_gdu8_read/1 -> Terminator_43/1
  ES011_u8_TasSent5SignalFault_st_gdu8_read/1 -> Terminator_44/1
  ES012_u8_HwAgCorrFault_st_gdu8_read/1 -> Terminator_45/1
  ES011_u8_TasSent5ProtFault_st_gdu8_read/1 -> Terminator_46/1
  ES012_u8_HwAgCalibrationFault_st_gdu8_read/1 -> Terminator_47/1
  ES001_u8_HwAgAOverLimFault_st_gdu8_read/1 -> Terminator_48/1
  ES010_u8_HwAgBOverLimFault_st_gdu8_read/1 -> Terminator_49/1
  MC005_u8_IMC1Fault_st_gdu8_read/1 -> Terminator_50/1
  MC005_u8_IMC2Fault_st_gdu8_read/1 -> Terminator_51/1
  ES008_u8_HiVltgErrorFault_st_gdu8_read/1 -> Terminator_52/1
  ES008_u8_HiVltgFatalErrorFault_st_gdu8_read/1 -> Terminator_53/1
  ES008_u8_LowVltgErrorFault_st_gdu8_read/1 -> Terminator_54/1
  ES008_u8_LowVltgFatalErrorFault_st_gdu8_read/1 -> Terminator_55/1
  ES008_u8_MotBrdgVltgADCFault_st_gdu8_read/1 -> Terminator_56/1
  ES008_u8_EPSSupplyVltgADCFault_st_gdu8_read/1 -> Terminator_57/1
  ES008_u8_SbcSupplyVltgADCFault_st_gdu8_read/1 -> Terminator_58/1
  ES008_u8_VltgCorrErrorSlightFault_st_gdu8_read/1 -> Terminator_59/1
  ES008_u8_VltgCorrErrorFatalFault_st_gdu8_read/1 -> Terminator_60/1
  ES007_u8_TempNTC1Fault_st_gdu8_read/1 -> Terminator_61/1
  ES007_u8_TempNTC2Fault_st_gdu8_read/1 -> Terminator_62/1
  ES007_u8_TempNTCCorrFault_st_gdu8_read/1 -> Terminator_63/1
  MF004_u8_ThermalProtectFault_st_gdu8_read/1 -> Terminator_64/1
  MC005_u8_IPCHeartBeatSignalFault_st_gdu8_read/1 -> Terminator_65/1
  MC001_u8_VCANBusoff_st_gdu8_read/1 -> Terminator_66/1
  MC001_u8_PrivateCANFault_st_gdu8_read/1 -> Terminator_67/1
  MC001_u8_LDCUMsgMissingFault_st_gdu8_read/1 -> Terminator_68/1
  MC001_u8_ESPMsgMissingFault_st_gdu8_read/1 -> Terminator_69/1
  MC001_u8_CDCUMsgMissingFault_st_gdu8_read/1 -> Terminator_70/1
  MC001_u8_MFSMsgMissingFault_st_gdu8_read/1 -> Terminator_71/1
  MC001_u8_XPUMsgMissingFault_st_gdu8_read/1 -> Terminator_72/1
  MC001_u8_DPBMsgMissingFault_st_gdu8_read/1 -> Terminator_73/1
  MC001_u8_XPUMsg1E2EFault_st_gdu8_read/1 -> Terminator_74/1
  MC001_u8_ESPMsg1E2EFault_st_gdu8_read/1 -> Terminator_75/1
  MC001_u8_MFSMsg1E2EFault_st_gdu8_read/1 -> Terminator_76/1
  MC001_u8_LDCUMsg1E2EFault_st_gdu8_read/1 -> Terminator_77/1
  MC001_u8_CDCUMsg1E2EFault_st_gdu8_read/1 -> Terminator_78/1
  MC001_u8_LDCUMsg2E2EFault_st_gdu8_read/1 -> Terminator_79/1
  MC001_u8_ESPMsg2E2EFault_st_gdu8_read/1 -> Terminator_80/1
  MC001_u8_LDCUMsg3E2EFault_st_gdu8_read/1 -> Terminator_81/1
  MC001_u8_DPBMsg1E2EFault_st_gdu8_read/1 -> Terminator_82/1
  MC001_u8_XPUSignal1Fault_st_gdu8_read/1 -> Terminator_83/1
  MC001_u8_ESPSignal1Fault_st_gdu8_read/1 -> Terminator_84/1
  MC001_u8_MFSSignal1Fault_st_gdu8_read/1 -> Terminator_85/1
  MC001_u8_ESPSignal2Fault_st_gdu8_read/1 -> Terminator_86/1
  MC001_u8_ESPSignal3Fault_st_gdu8_read/1 -> Terminator_87/1
  MC001_u8_ESPSignal4Fault_st_gdu8_read/1 -> Terminator_88/1
  MC001_u8_LDCUSignal1Fault_st_gdu8_read/1 -> Terminator_89/1
  MC001_u8_DPBSignal1Fault_st_gdu8_read/1 -> Terminator_90/1
  MC001_u8_LDCUSignal2Fault_st_gdu8_read/1 -> Terminator_91/1
  MC001_u8_LDCUSignal3Fault_st_gdu8_read/1 -> Terminator_92/1
  MC001_u8_LDCUSignal4Fault_st_gdu8_read/1 -> Terminator_93/1
  SF035_u8_ChatterRednAssiFault_st_gdu8_read/1 -> Terminator_94/1
  SF022_u8_EOTNotLearnedFault_st_gdu8_read/1 -> Terminator_95/1
  SF026_u8_MecFricTooHiFault_st_gdu8_read/1 -> Terminator_96/1
  SF010_u8_SysStErrorFault_st_gdu8_read/1 -> Terminator_97/1
  ES003_u8_MotAgCalibrationFault_st_gdu8_read/1 -> Terminator_98/1
  SF012_u8_RCOModlErrorFault_st_gdu8_read/1 -> Terminator_99/1
  SF010_u8_SysStSyncErrorFault_st_gdu8_read/1 -> Terminator_100/1
  MF010_u8_MotStallLimitFault_st_gdu8_read/1 -> Terminator_101/1
  Ground_1/1 -> SF020_u8_SysFaultLevel_UL_gdu8_write/1
  Ground_2/1 -> SF020_u8_SysFaultStatusArray_UL_ArrayU32_write/1
  Ground_3/1 -> SF020_f32_SysAssDegradeFactor_UL_gdf32_write/1
  Ground_4/1 -> SF020_u8_MotCtrlAssistType_UL_gdu8_write/1
  Signal Copy/1 -> Terminator_1/1

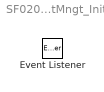
== system SF020_SysFaultMngt/SF020_SysFaultMngt_Init ==
  Event Listener : EventListener  EventName=reset
